simulink model "UKF_Test"  (Simulink 9.0)
settings: Solver=ode4  StartTime=start_time  StopTime=stop_time  FixedStep=T_s  RelTol=1e-3  EnableMultiTasking=on
InitFcn:
  | init;
values from neighbouring files (symbols this model uses):
  T_s = model_parameters    [fstate.m]    (also in init.m = 0.0246)
libraries: dspsrcs4 x4
settings Model: LogicAnalyzerSignalOrdering=8ea762f0-fdaa-4d87-bee0-5db8bb381934,8849105a-1fa5-46c6-a087-1fc218fa0193,543442ae-4262-4358-a8de-c879cbc837b4,f37346fd-2075-4366-98d6-c49f7c685a94,617cba3a-ba40-4c7e-a0d3-838b0de1e4b1,707e89eb-2f58-4970-a176-5050bb12b326,8dcce648-08f4-4894-909a-da55f651ca11,6c20086e-ca58-42b9-b8c5-20be5936ff04,ea6cb4eb-9a0a-491a-bb55-a1b7ffccddfb  SuppressorTable=22 serialization::archive 11 0 6 0 0 0 0 0  Creator=lueken  LastModifiedBy=jules-pc
settings DataIOCC: LimitDataPoints=on
settings GRTTargetCC: GeneratePreprocessorConditionals=Disable all
settings ConfigComp: CovSFcnEnable=off

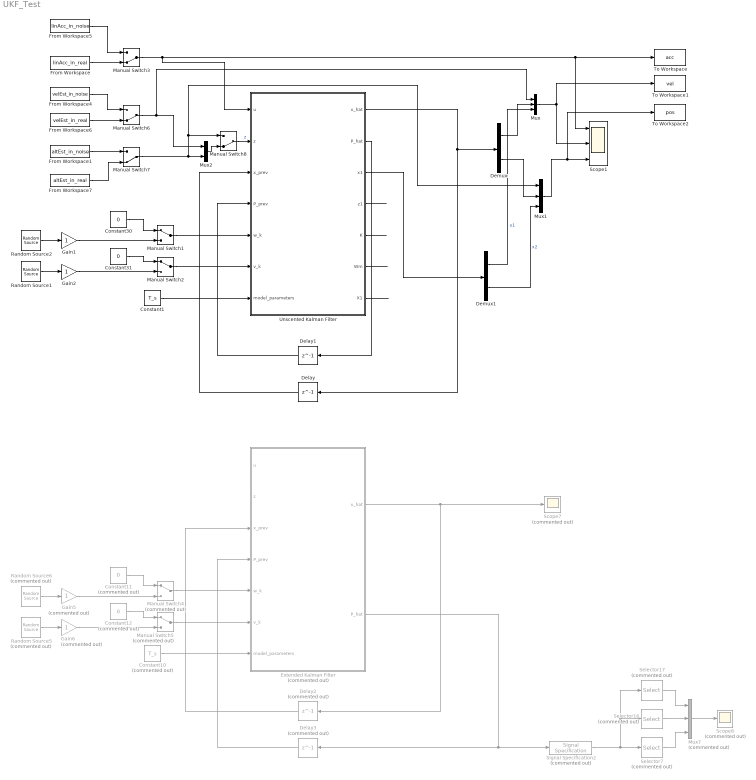
== system UKF_Test ==
  Constant1 : Constant  Value=T_s
  Constant10 : Constant  Commented=on  Value=T_s
  Constant11 : Constant  Commented=on  Value=0
  Constant12 : Constant  Commented=on  Value=0
  Constant30 : Constant  Value=0
  Constant31 : Constant  Value=0
  Delay : Delay  DelayLength=1  InitialCondition=[0 0]  InputProcessing=Inherited
  Delay1 : Delay  DelayLength=1  InitialCondition=[1 0;0 1]  InputProcessing=Inherited
  Delay2 : Delay  Commented=on  DelayLength=1  InitialCondition=[0 0 0]  InputProcessing=Inherited
  Delay3 : Delay  Commented=on  DelayLength=1  InitialCondition=eye(3)  InputProcessing=Inherited
  Demux : Demux  Outputs=2
  Demux1 : Demux  Outputs=2
  Extended Kalman Filter : MATLAB Function  Commented=on  TreatAsAtomicUnit=on
  From Workspace : FromWorkspace  VariableName=linAcc_in_real
  From Workspace1 : FromWorkspace  VariableName=altEst_in_noise
  From Workspace4 : FromWorkspace  VariableName=velEst_in_noise
  From Workspace5 : FromWorkspace  VariableName=linAcc_in_noise
  From Workspace6 : FromWorkspace  VariableName=velEst_in_real
  From Workspace7 : FromWorkspace  VariableName=altEst_in_real
  Gain1 : Gain
  Gain2 : Gain
  Gain5 : Gain  Commented=on
  Gain6 : Gain  Commented=on
  Manual Switch1 : ManualSwitch
  Manual Switch2 : ManualSwitch
  Manual Switch{3,6..8} (4 alike) : ManualSwitch  CurrentSetting=0
  Manual Switch4 : ManualSwitch  Commented=on
  Manual Switch5 : ManualSwitch  Commented=on
  Mux : Mux  Inputs=3
  Mux1 : Mux  Inputs=3
  Mux2 : Mux  Inputs=2
  Mux7 : Mux  Commented=on  Inputs=3
  Random Source1 : dspsrcs4/Random Source  SrcType=Gaussian  NormMethod=Ziggurat  CltLength=12  MinVal=0  MaxVal=1  MeanVal=0  VarVal=0.01^2  RepMode=Not repeatable  rawSeed=1  IsInherit=off  SampMode=Continuous  SampTime=1  SampFrame=1  DataType=Double  OutComplex=Real  OutputFrames=on
  Random Source2 : dspsrcs4/Random Source  SrcType=Gaussian  NormMethod=Ziggurat  CltLength=12  MinVal=0  MaxVal=1  MeanVal=0  VarVal=0.01^2  RepMode=Not repeatable  rawSeed=1  IsInherit=off  SampMode=Continuous  SampTime=1  SampFrame=1  DataType=Double  OutComplex=Real  OutputFrames=on
  Random Source5 : dspsrcs4/Random Source  Commented=on  SrcType=Gaussian  NormMethod=Ziggurat  CltLength=12  MinVal=0  MaxVal=1  MeanVal=0  VarVal=0.01^2  RepMode=Not repeatable  rawSeed=1  IsInherit=off  SampMode=Continuous  SampTime=1  SampFrame=1  DataType=Double  OutComplex=Real  OutputFrames=on
  Random Source6 : dspsrcs4/Random Source  Commented=on  SrcType=Gaussian  NormMethod=Ziggurat  CltLength=12  MinVal=0  MaxVal=1  MeanVal=0  VarVal=0.01^2  RepMode=Not repeatable  rawSeed=1  IsInherit=off  SampMode=Continuous  SampTime=1  SampFrame=1  DataType=Double  OutComplex=Real  OutputFrames=on
  Scope1 : Scope  NumInputPorts=3
  Scope7 : Scope  Commented=on
  Scope8 : Scope  Commented=on
  Selector16 : Selector  Commented=on  NumberOfDimensions=2  InputPortWidth=[3 3]  IndexOptions=Index vector (dialog),Index vector (dialog)  Indices=[2],[2]  OutputSizes=1,1
  Selector17 : Selector  Commented=on  NumberOfDimensions=2  InputPortWidth=[3 3]  IndexOptions=Index vector (dialog),Index vector (dialog)  Indices=[1],[1]  OutputSizes=1,1
  Selector7 : Selector  Commented=on  NumberOfDimensions=2  InputPortWidth=[3 5]  IndexOptions=Index vector (dialog),Index vector (dialog)  Indices=[3],[3]  OutputSizes=1,1
  Signal Specification2 : SignalSpecification  Commented=on  Dimensions=[3 3]
  To Workspace : ToWorkspace  VariableName=acc  SaveFormat=Timeseries  SampleTime=-1
  To Workspace1 : ToWorkspace  VariableName=vel  SaveFormat=Timeseries  SampleTime=-1
  To Workspace2 : ToWorkspace  VariableName=pos  SaveFormat=Timeseries  SampleTime=-1
  Unscented Kalman Filter : MATLAB Function  TreatAsAtomicUnit=on
  wires:
  Random Source1/1 -> Gain2/1
  Random Source2/1 -> Gain1/1
  Delay/1 -> Unscented Kalman Filter/3(x_prev)
  Delay1/1 -> Unscented Kalman Filter/4(P_prev)
  Unscented Kalman Filter/1(x_hat) -> Delay/1, Demux/1
  Constant30/1 -> Manual Switch1/1
  Constant31/1 -> Manual Switch2/1
  Gain2/1 -> Manual Switch2/2
  Manual Switch2/1 -> Unscented Kalman Filter/6(v_k)
  Manual Switch1/1 -> Unscented Kalman Filter/5(w_k)
  Gain1/1 -> Manual Switch1/2
  Constant1/1 -> Unscented Kalman Filter/7(model_parameters)
  Random Source5/1 -> Gain6/1
  Random Source6/1 -> Gain5/1
  Delay2/1 -> Extended Kalman Filter/3(x_prev)
  Delay3/1 -> Extended Kalman Filter/4(P_prev)
  Constant11/1 -> Manual Switch4/1
  Constant12/1 -> Manual Switch5/1
  Gain6/1 -> Manual Switch5/2
  Manual Switch5/1 -> Extended Kalman Filter/6(v_k)
  Manual Switch4/1 -> Extended Kalman Filter/5(w_k)
  Gain5/1 -> Manual Switch4/2
  Extended Kalman Filter/2(P_hat) -> Delay3/1, Signal Specification2/1
  Signal Specification2/1 -> Selector17/1, Selector16/1, Selector7/1
  Selector16/1 -> Mux7/2
  Mux7/1 -> Scope8/1
  Selector17/1 -> Mux7/1
  Selector7/1 -> Mux7/3
  Constant10/1 -> Extended Kalman Filter/7(model_parameters)
  Extended Kalman Filter/1(x_hat) -> Scope7/1, Delay2/1
  Manual Switch7/1 -> Manual Switch8/1, Mux1/1, Mux2/2
  Demux/1 -> Mux/2
  Manual Switch6/1 -> Mux/1, Mux2/1
  Mux/1 -> To Workspace1/1, Scope1/2
  Demux/2 -> Mux1/2
  Mux1/1 -> To Workspace2/1, Scope1/3
  Unscented Kalman Filter/3(x1) -> Demux1/1
  Manual Switch3/1 -> Unscented Kalman Filter/1(u), To Workspace/1, Scope1/1
  From Workspace4/1 -> Manual Switch6/1
  Mux2/1 -> Manual Switch8/2
  From Workspace5/1 -> Manual Switch3/1
  From Workspace/1 -> Manual Switch3/2
  From Workspace6/1 -> Manual Switch6/2
  From Workspace1/1 -> Manual Switch7/1
  From Workspace7/1 -> Manual Switch7/2
  Manual Switch8/1 -> Unscented Kalman Filter/2(z)  "z"
  Unscented Kalman Filter/2(P_hat) -> Delay1/1
  Demux1/1 -> Mux/3  "x1"
  Demux1/2 -> Mux1/3  "x2"
  Unscented Kalman Filter/4(z1) -> ?
  Unscented Kalman Filter/5(K) -> ?
  Unscented Kalman Filter/6(Wm) -> ?
  Unscented Kalman Filter/7(X1) -> ?

== matlab function Extended Kalman Filter ==
  data: u input double; z input double; x_hat output double; x_prev input double; P_prev input double; w_k input double; v_k input double; P_hat output double; model_parameters input double
function [x_hat,P_hat]=ekf(u,z,x_prev,P_prev,w_k,v_k,model_parameters)
% EKF   Extended Kalman Filter for nonlinear dynamic systems
% [x, P] = ekf(f,x,P,h,z,Q,R) returns state estimate, x and state covariance, P 
% for nonlinear dynamic system:
%           x_k+1 = f(x_k) + w_k
%           z_k   = h(x_k) + v_k
% where w ~ N(0,Q) meaning w is gaussian noise with covariance Q
%       v ~ N(0,R) meaning v is gaussian noise with covariance R
% Inputs:   f: function handle for f(x)
%           x: "a priori" state estimate
%           P: "a priori" estimated state covariance
%           h: fanction handle for h(x)
%           z: current measurement
%           Q: process noise covariance 
%           R: measurement noise covariance
% Output:   x: "a posteriori" state estimate
%           P: "a posteriori" state covariance
%}
% By Yi Cao at Cranfield University, 02/01/2008
%
N_x=numel(x_prev);      %numer of states
q=numel(z);             %numer of measurements

m=0.1;                  %std of process 
r=0.01;                 %std of measurement
Q=m^2*eye(N_x);         %covariance of process
R=r^2;                  %covariance of measurement  

[x1,A]=jaccsd(@fstate,x_prev,u,w_k,model_parameters);    %nonlinear update and linearization at current state
P=A*P_prev*A'+Q;                 %partial update
[z1,H]=jaccsd(@hmeas,x1,u,v_k,model_parameters);    %nonlinear measurement and linearization
P12=P*H';                   %cross covariance
% K=P12*inv(H*P12+R);       %Kalman filter gain
% x=x1+K*(z-z1);            %state estimate
% P=P-K*P12';               %state covariance matrix
R=chol(H*P12+R);            %Cholesky factorization
U=P12/R;                    %K=U/R'; Faster because of back substitution
x_hat=x1+U*(R'\(z-z1));         %Back substitution to get state update
P_hat=P-U*U';                   %Covariance update, U*U'=P12/R/R'*P12'=K*P12.


% hold off;
% coder.extrinsic('error_ellipse'); 
% error_ellipse(P_prev(1:2,1:2),x_prev);
% hold on;
% error_ellipse(P(1:2,1:2),x1,'style','r');
% axis([-100 100 0 100])

== matlab function Unscented Kalman Filter ==
  data: u input double; z input double; x_hat output double; x_prev input double; P_prev input double; w_k input double; v_k input double; P_hat output double; model_parameters input double; x1 output double; z1 output double; K output double; Wm output double; X1 output double
function [x_hat,P_hat,x1,z1,K,Wm,X1]=ukf(u,z,x_prev,P_prev,w_k,v_k,model_parameters)
% UKF   Unscented Kalman Filter for nonlinear dynamic systems
% [x, P] = ukf(f,x,P,h,z,Q,R) returns state estimate, x and state covariance, P 
% for nonlinear dynamic system (for simplicity, noises are assumed as additive):
%           x_k+1 = f(x_k, u_k) + w_k
%           z_k   = h(x_k, u_k) + v_k
% where w ~ N(0,Q) meaning w is gaussian noise with covariance Q
%       v ~ N(0,R) meaning v is gaussian noise with covariance R
% Inputs:   f: function handle for f(x)
%           x: "a priori" state estimate
%           P: "a priori" estimated state covariance
%           h: fanction handle for h(x)
%           z: current measurement
%           Q: process noise covariance 
%           R: measurement noise covariance
% Output:   x: "a posteriori" state estimate
%           P: "a posteriori" state covariance
%
% Reference: Julier, SJ. and Uhlmann, J.K., Unscented Filtering and
% Nonlinear Estimation, Proceedings of the IEEE, Vol. 92, No. 3,
% pp.401-422, 2004. 
%
% By Yi Cao at Cranfield University, 04/01/2008
%
N_x=numel(x_prev);      %number of states
N_z=numel(z);             %number of measurements

%% Simulation parameters
Q=[0.0024 0;...
    0 0.1183];         %covariance of process
R=[3.7195 0;...
  0     0.34];           %covariance of measurement  

Q=[2.747862641657714e-07 8.005915795518623e-05;8.005915795518623e-05 0.103200057112597];
R=[0.000103786356167880 0.00190427431408450;0.00190427431408450 0.130583830229682];
%% real parameters
% m=0.001;                %std of process 
% r=0.001;                    %std of measurement
% M=m^2*eye(N_x);       %covariance of process
% R=r*eye(N_z);           %covariance of measurement  
% R=[1 0;...
%     0 0,001];           %covariance of measurement  

alpha=0.001;            %small positive value ([10^-4...1])
kappa=3-N_x;                %constant, usually 0 or 3-N_x
beta=2;                 %2 optimal for Gaussian Distribution
lambda=alpha^2*(N_x+kappa)-N_x;             %scaling parameter
c=N_x+lambda;                               %scaling parameter
Wm=[lambda/c 0.5/c+zeros(1,2*N_x)];         %weights for means
Wc=Wm;
Wc(1)=Wc(1)+(1-alpha^2+beta);               %weights for covariancee
c=sqrt(c);
X=sigmas(x_prev,P_prev,c);                  %sigma points around x

%unscented transformation of process (Gl. (4.13)-(4.16))
[x1,X1,P1,X2]=ut(@fstate,X,u,Wm,Wc,N_x,Q,w_k,model_parameters);          
X1=sigmas(x1,P1,c); % Gl. (4.9) (Paper (7.56))
%unscented transformation of measurments (Gl. (4.18)-(4.21))
[z1,Z1,P2,Z2]=ut(@hmeas,X1,0,Wm,Wc,N_z,R,v_k,model_parameters);       
%transformed cross-covariance GL. (4.22)
P12=X2*diag(Wc)*Z2';   

K=P12*inv(P2);%P2\P12;%*inv(P2); Gl.(4.23)
x_hat=x1+K*(z-z1);                              %state update Gl.(4.24)
P_hat=P1-K*P2*K';                               %covariance update GL.(4.25)


% hold off;
% coder.extrinsic('error_ellipse'); 
% error_ellipse(P_prev(1:2,1:2),x_prev);
% hold on;
% error_ellipse(P1(1:2,1:2),x1,'style','r');
% plot(X(1,:),X(2,:),'x')
% plot(X1(1,:),X1(2,:),'xr')
% %axis([-100 100 0 100])
